simulink model "Battery_model"  (R2023b)
settings: Solver=FixedStepDiscrete  StartTime=0.0  StopTime=30000  RelTol=1e-3
values from neighbouring files (symbols this model uses):
  cf = 17e-6    (= 1.7e-05)    [Parameters.m]
  Kii_d = 100    [Parameters.m]
  Kii_dc = 0.003    [Parameters.m]
  Kii_q = 100    [Parameters.m]
  Kiv_dc = 10    [Parameters.m]
  Kpi_d = 1    [Parameters.m]
  Kpi_dc = 0.1    [Parameters.m]
  Kpi_q = 1    [Parameters.m]
  Kpv_dc = 30    [Parameters.m]
  lf = 1e-3    (= 0.001)    [Parameters.m]
  rf = 0    [Parameters.m]
  T_camp = 1    [Parameters.m]
  Ts_p = 80.0e-06    (= 8e-05)    [Parameters.m]
  Ts_Power = 80.0e-06    (= 8e-05)    [Parameters.m]
  V_ref_dc_link = 750    [Parameters.m]
undefined symbols (not defined in the file or in its folder): Ion, Lithium
libraries: spsRMSLib x9, spsThreePhaseVIMeasurementLib x5, slpidlib x4, spsabctodq0Lib x3, spsVoltageMeasurementLib x3, spsPower3phInstantaneousLib x3, spsPLLLib x3, spsTHDLib x3, simulink x2, spsCurrentMeasurementLib x2, spsThreePhaseSeriesRLCBranchLib x2, spsBatteryLib x1
settings Model: SimulationMode=accelerator  Creator=robby  LastModifiedBy=alessandroarmellin
settings SolverCC: AlgebraicLoopSolver=TrustRegion
settings DataIOCC: InitialState=out.xFinal  SaveFinalState=on  SaveOperatingPoint=on
settings ModelReferenceCC: EnableRefExpFcnMdlSchedulingChecks=on
settings RTWCC: DLArmComputeVersion=19.05

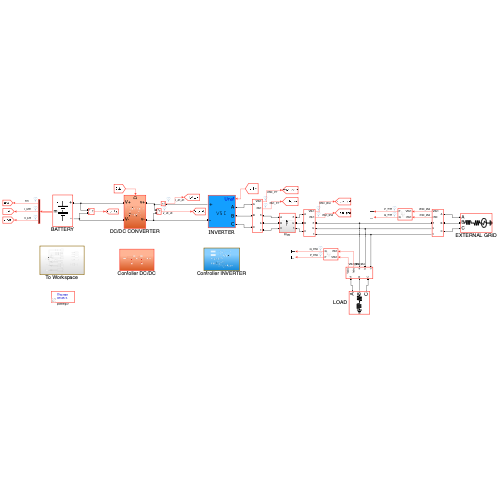
[thumbnail: Simulink's stored preview of the top-level diagram]
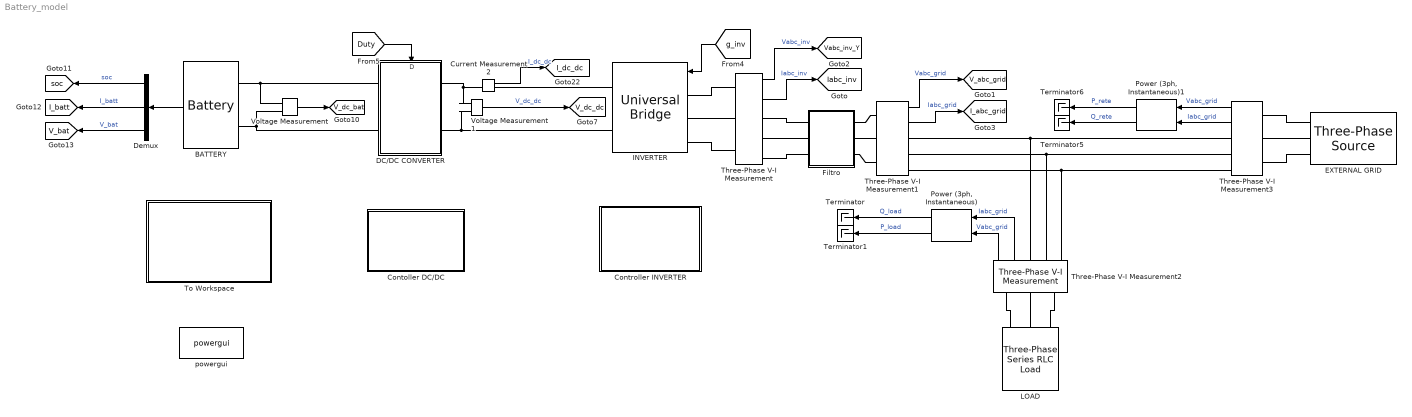
== system Battery_model ==
  BATTERY : spsBatteryLib/Battery  BatType=Lithium-Ion  ShowTempParam=off  ThermalPreset=no  ShowAgeParam=off  NomV=V_batt_nom  NomQ=Cap_bat_nom  SOC=soc_tot  Batt_Tr=1  PresetModel=on  MaxQ=200  MinV=465  FullV=721.672  Dis_rate=86.9565  R=0.031  Normal_OP=180.8696  expZone="[669.8392      9.826087]"  current=[6.5 13 32.5]  Units=Time  Tci=20  NomT=20  T2=-30  MaxQ2=4.8  FullV2=7.1  Normal_OP2=5.655  expZone2="[6.58           1]"  Rca=0.6  ti=2000  Dp=0  Neq0=0  Tsim=1e6  Ta1=25  Qeol=5.4*0.9  Reol=0.013333*1.2  Char_age=[2.3478, 3]  Dis_age=[2.3478, 10]  N1=1500  N2=10500  N3=1000  N4=1400  Ta2=45  N5=950
  Contoller DC/DC : Subsystem
  Controller INVERTER : Subsystem
  Current Measurement2 : spsCurrentMeasurementLib/Current Measurement  PhasorSimulation=off  OutputType=Complex  PSBequivalent=0
  DC/DC CONVERTER : Subsystem
      settings: PortSchema="{\"entries\":[{\"content\":{\"sides\":[{\"content\":{\"connectorIds\":[\"LConn1\",\"LConn2\"]},\"type\":\"ConnectorPlacement.EquallySpacedRectSide\",\"uuid\":\"1063a80c-0db9-4e6a-b0a1-ad7a8a9cb9ed\"},{\"content\":{\"connectorIds\":[\"RConn1\",\"RConn2\"],\"side\":\"RIGHT\"},\"type\":\"ConnectorPlacement.EquallySpacedRectSide\",\"uuid\":\"d09a7538-6c2e-450d-96ff-912ee6979d92\"},{\"content\":{\"connectorIds\":[\"In1\"],\"side\":\"TOP\"},\"type\":\"ConnectorPlacement.EquallySpacedRectSide\",\"uuid\":\"7f294bc1-8c9a-4b69-a306-35098527c416\"},{\"content\":{\"connectorIds\":[],\"side\":\"HIDDEN\"},\"type\":\"ConnectorPlacement.EquallySpacedRectSide\",\"uuid\":\"5677a460-882c-466a-84c4-3fc7d1866fb0\"}]},\"type\":\"ConnectorPlacement.EquallySpacedConnector\",\"uuid\":\"dc710a20-86db-486e-80ec-dfab0fa59d77\"}],\"packageUris\":[\"http://schema.mathworks.com/mf0/Connector/R2020b\"],\"version\":\"1.0\"}"
  Demux : Demux  Outputs=3
  EXTERNAL GRID : spsThreePhaseSourceLib/Three-Phase Source  InternalConnection=Yg  VoltagePhases=off  Voltage=400  PhaseAngle=0  Voltage_phases=[25e3 25e3 25e3]/sqrt(3)  PhaseAngles_phases=[0 -120 +120]  Frequency=50  NonIdealSource=on  SpecifyImpedance=off  Resistance=0.1  Inductance=1e-6  ShortCircuitLevel=1e6  BaseVoltage=400  XRratio=7  BusType=swing  Pref=10e3  Qref=0  Prefabc=[10e3, 10e3, 10e3]  Qrefabc=[0, 0, 0]  Qmin=-inf  Qmax=inf
  Filtro : Subsystem
  INVERTER : spsUniversalBridgeLib/Universal Bridge  Arms=3  SnubberResistance=1e5  SnubberCapacitance=inf  Device=Average-model based VSC  Ron=1e-3  Lon=0  ForwardVoltages="[  0  0  ]"  ForwardVoltage=0  GTOparameters=[ 10e-6 , 20e-6 ]  IGBTparameters=[ 1e-6 , 2e-6 ]  Measurements=None  Measurements_2=None  converterType=Rectifier
  LOAD : spsThreePhaseSeriesRLCLoadLib/Three-Phase Series RLC Load  LConnTagsString=A|B|C  Configuration=Y (grounded)  NominalVoltage=400  Vabc=[1e3 1e3 1e3]  Vabcp=[1e3 1e3 1e3]  NominalFrequency=50  UnbalancedPower=off  ActivePower=2000  InductivePower=150  CapacitivePower=0  Pabc=[10e3 9e3 11e3]  QLabc=[100 90 110]  QCabc=[100 90 110]  Pabcp=[10e3 9e3 11e3]  QLabcp=[100 90 110]  QCabcp=[100 90 110]  Measurements=None  LoadType=constant Z
  "Power (3ph, Instantaneous)" : spsPower3phInstantaneousLib/Power (3ph, Instantaneous)
  "Power (3ph, Instantaneous)1" : spsPower3phInstantaneousLib/Power (3ph, Instantaneous)
  Terminator{,1,5..6} (4 alike) : Terminator
  Three-Phase V-I Measurement{,1..3} (4 alike) : spsThreePhaseVIMeasurementLib/Three-Phase V-I Measurement  VoltageMeasurement=phase-to-ground  SetLabelV=off  LabelV=Vabc_cond  Vpu=off  VpuLL=off  CurrentMeasurement=yes  SetLabelI=off  LabelI=Iabc_cond  Ipu=off  Pbase=100e6  Vbase=500e3  OutputType=Complex  PhasorSimulation=off  PSBequivalent=0
  To Workspace : Subsystem
  Voltage Measurement : spsVoltageMeasurementLib/Voltage Measurement  PhasorSimulation=off  OutputType=Complex  PSBequivalent=0
  Voltage Measurement1 : spsVoltageMeasurementLib/Voltage Measurement  PhasorSimulation=off  OutputType=Complex  PSBequivalent=0
  powergui : spspowerguiLib/powergui  Priority=1  SimulationMode=Discrete  SampleTime=Ts_Power  frequency=60  Iterations=50  frequencyindice=50  Pbase=100e6  ErrMax=1e-4  UnitsV=kV  UnitsW=MW  buscounter=1  FunctionMessages=off  echomessages=off  EnableUseOfTLC=off  CurrentSourceSwitches=off  DisableSnubberDevices=off  DisableRonSwitches=off  DisableVfSwitches=off  DisplayEquations=off  AutomaticDiscreteSolvers=off  SolverType=Tustin/Backward Euler (TBE)  Interpol=off  ExternalGateDelay=off  methode=off  Ts=100  x0status=blocks  SPID=on  SwTol=0  HookPort=off  NonlinearTolerance=1e-4  nMaxIteration=100  ContinueOnMaxIteration=off  RestoreLinks=warning  ResistiveCurrentMeasurement=off  Frange=[0:2:500]  Ylog=off  Xlog=on  ShowGrid=off  save=off  variable=ZData  structure=0  ZoomFFT=off  StartTime=0.0  cycles=1  DisplayStyle=1  fundamental=60  FreqAxis=off  MaxFrequency=1000  frequencyindicesteady=1  RmsSteady=1  display=off
  tag scope: I_abc_grid=global, I_batt=global, I_dc_dc=global, Iabc_inv=global, V_abc_grid=global, V_bat=global, V_dc_bat=global, V_dc_dc=global, Vabc_inv_Y=global, soc=global
  wires:
  Three-Phase V-I Measurement/1 -> [Vabc_inv_Y]  "Vabc_inv"
  Three-Phase V-I Measurement/2 -> [Iabc_inv]  "Iabc_inv"
  Voltage Measurement1/1 -> [V_dc_dc]  "V_dc_dc"
  Current Measurement2/1 -> [I_dc_dc]  "I_dc_dc"
  [g_inv] -> INVERTER/1
  [Duty] -> DC/DC CONVERTER/1(D)
  BATTERY/1 -> Demux/1
  Demux/1 -> [soc]  "soc"
  Demux/2 -> [I_batt]  "I_batt"
  Demux/3 -> [V_bat]  "V_bat"
  Three-Phase V-I Measurement1/1 -> [V_abc_grid]  "Vabc_grid"
  Three-Phase V-I Measurement1/2 -> [I_abc_grid]  "Iabc_grid"
  Voltage Measurement/1 -> [V_dc_bat]
  Three-Phase V-I Measurement2/1 -> "Power (3ph, Instantaneous)"/1  "Vabc_grid"
  Three-Phase V-I Measurement2/2 -> "Power (3ph, Instantaneous)"/2  "Iabc_grid"
  "Power (3ph, Instantaneous)"/2 -> Terminator/1  "Q_load"
  "Power (3ph, Instantaneous)"/1 -> Terminator1/1  "P_load"
  "Power (3ph, Instantaneous)1"/1 -> Terminator6/1  "P_rete"
  "Power (3ph, Instantaneous)1"/2 -> Terminator5/1  "Q_rete"
  Three-Phase V-I Measurement3/2 -> "Power (3ph, Instantaneous)1"/2  "Iabc_grid"
  Three-Phase V-I Measurement3/1 -> "Power (3ph, Instantaneous)1"/1  "Vabc_grid"
  connections:
  Three-Phase V-I Measurement/LConn3 -- INVERTER/LConn3
  Three-Phase V-I Measurement/LConn2 -- INVERTER/LConn2
  Current Measurement2/RConn1 -- INVERTER/RConn1
  Current Measurement2/LConn1 -- Voltage Measurement1/LConn1 -- DC/DC CONVERTER/RConn1
  Voltage Measurement1/LConn2 -- INVERTER/RConn2 -- DC/DC CONVERTER/RConn2
  BATTERY/LConn1 -- Voltage Measurement/LConn1 -- DC/DC CONVERTER/LConn1
  Voltage Measurement/LConn2 -- BATTERY/LConn2 -- DC/DC CONVERTER/LConn2
  Filtro/LConn3 -- Three-Phase V-I Measurement/RConn3
  Filtro/LConn2 -- Three-Phase V-I Measurement/RConn2
  Filtro/LConn1 -- Three-Phase V-I Measurement/RConn1
  INVERTER/LConn1 -- Three-Phase V-I Measurement/LConn1
  Three-Phase V-I Measurement1/RConn2 -- Three-Phase V-I Measurement3/RConn2 -- Three-Phase V-I Measurement2/RConn2
  Three-Phase V-I Measurement2/RConn1 -- Three-Phase V-I Measurement1/RConn1 -- Three-Phase V-I Measurement3/RConn1
  Three-Phase V-I Measurement2/RConn3 -- Three-Phase V-I Measurement1/RConn3 -- Three-Phase V-I Measurement3/RConn3
  Three-Phase V-I Measurement1/LConn2 -- Filtro/RConn2
  Three-Phase V-I Measurement1/LConn3 -- Filtro/RConn3
  Filtro/RConn1 -- Three-Phase V-I Measurement1/LConn1
  Three-Phase V-I Measurement2/LConn2 -- LOAD/LConn2
  Three-Phase V-I Measurement2/LConn1 -- LOAD/LConn1
  Three-Phase V-I Measurement2/LConn3 -- LOAD/LConn3
  EXTERNAL GRID/RConn2 -- Three-Phase V-I Measurement3/LConn2
  Three-Phase V-I Measurement3/LConn1 -- EXTERNAL GRID/RConn1
  Three-Phase V-I Measurement3/LConn3 -- EXTERNAL GRID/RConn3

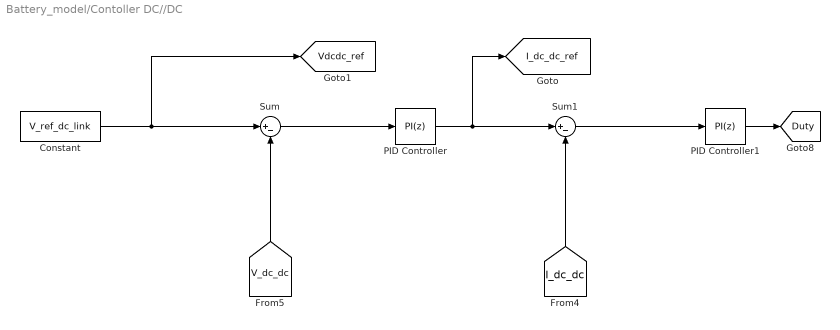
== system Battery_model/Contoller DC//DC ==
  Constant : Constant  Value=V_ref_dc_link
  PID Controller : slpidlib/PID Controller  Controller=PI  Form=Parallel  TimeDomain=Discrete-time  UseExternalTs=off  SampleTime=Ts_p  IntegratorMethod=Forward Euler  FilterMethod=Forward Euler  ControllerParametersSource=internal  P=Kiv_dc  I=Kpv_dc  UseKiTs=off  D=0  N=100  UseFilter=on  TunerSelectOption=Transfer Function Based (PID Tuner App)  InitialConditionSource=internal  InitialConditionForIntegrator=0  InitialConditionForFilter=0  DifferentiatorICPrevScaledInput=0  ExternalReset=none  TrackingMode=off  Kt=1  LimitOutput=off  SatLimitsSource=internal  UpperSaturationLimit=1  LowerSaturationLimit=-1  LinearizeAsGain=on  AntiWindupMode=none  Kb=1  LimitIntegrator=off  UpperIntegratorSaturationLimit=inf  LowerIntegratorSaturationLimit=-inf  POutMin=[]  POutMax=[]  IOutMin=[]  IOutMax=[]  DOutMin=[]  DOutMax=[]  NOutMin=[]  NOutMax=[]  SumOutMin=[]  SumOutMax=[]  SaturationOutMin=[]  SaturationOutMax=[]  PParamMin=[]  PParamMax=[]  IParamMin=[]  IParamMax=[]  DParamMin=[]  DParamMax=[]  NParamMin=[]  NParamMax=[]  KbParamMin=[]  KbParamMax=[]  KtParamMin=[]  KtParamMax=[]  KbOutMin=[]  KbOutMax=[]  KtOutMin=[]  KtOutMax=[]  IntegratorOutMin=[]  IntegratorOutMax=[]  FilterOutMin=[]  FilterOutMax=[]  SumI1OutMin=[]  SumI1OutMax=[]  SumI2OutMin=[]  SumI2OutMax=[]  SumI3OutMin=[]  SumI3OutMax=[]  SumI4OutMin=[]  SumI4OutMax=[]  SumDOutMin=[]  SumDOutMax=[]  DifferentiatorOutMin=[]  DifferentiatorOutMax=[]  FilterDiffOutCoefMin=[]  FilterDiffOutCoefMax=[]  ReciprocalOutMin=[]  ReciprocalOutMax=[]  SumDenOutMin=[]  SumDenOutMax=[]  SumNumOutMin=[]  SumNumOutMax=[]  DivideOutMin=[]  DivideOutMax=[]  UdiffTsProdOutMin=[]  UdiffTsProdOutMax=[]  NTsProdOutMin=[]  NTsProdOutMax=[]  UintegralTsProdOutMin=[]  UintegralTsProdOutMax=[]  UngainTsProdOutMin=[]  UngainTsProdOutMax=[]  ClampingZeroOutDataTypeStr=Inherit: Inherit via back propagation  ClampingZeroOutMin=[]  ClampingZeroOutMax=[]  FilterDenConstantOutDataTypeStr=Inherit: Inherit via back propagation  FilterDenConstantOutMin=[]  FilterDenConstantOutMax=[]  PCopyOutDataTypeStr=Inherit: Inherit via back propagation  PCopyOutMin=[]  PCopyOutMax=[]  NCopyOutDataTypeStr=Inherit: Inherit via back propagation  NCopyOutMin=[]  NCopyOutMax=[]  IntegratorContinuousStateAttributes=''  IntegratorStateMustResolveToSignalObject=off  IntegratorRTWStateStorageClass=Auto  FilterContinuousStateAttributes=''  FilterStateMustResolveToSignalObject=off  FilterRTWStateStorageClass=Auto  ParallelPVariant=InternalParameters  IdealPVariant=Disabled  IVariant=InternalParameters  DVariant=Disabled  IntegratorVariant=Discrete  SatVariant=Disabled  AWVariant=Passthrough  PCopyVariant=Disabled  TRVariant=Disabled  FdbkBlocksVariant=Forward  IdealPFdbkVariant=Disabled  SatFdbkVariant=Disabled  DerivativeFilterVariant=Disabled  NVariant=Disabled  NCopyVariant=Disabled_SignalSpec  FilterICVariant=Disabled  IntegratorICVariant=InternalICs  ExternalResetVariant=Disabled  TRSumVariant=Passthrough  SumFdbkVariant=Disabled  SumVariant=Sum_PI  TsampFilterVariant=InternalTs  TsampNgainVariant=Passthrough  TsampIntegralVariant=Disabled_SignalSpec  ExternalSaturationOutDataTypeStr=Inherit: Same as second input
  PID Controller1 : slpidlib/PID Controller  Controller=PI  Form=Parallel  TimeDomain=Discrete-time  UseExternalTs=off  SampleTime=Ts_p  IntegratorMethod=Forward Euler  FilterMethod=Forward Euler  ControllerParametersSource=internal  P=Kii_dc  I=Kpi_dc  UseKiTs=off  D=0  N=100  UseFilter=on  TunerSelectOption=Transfer Function Based (PID Tuner App)  InitialConditionSource=internal  InitialConditionForIntegrator=0  InitialConditionForFilter=0  DifferentiatorICPrevScaledInput=0  ExternalReset=none  TrackingMode=off  Kt=1  LimitOutput=off  SatLimitsSource=internal  UpperSaturationLimit=1  LowerSaturationLimit=-1  LinearizeAsGain=on  AntiWindupMode=none  Kb=1  LimitIntegrator=off  UpperIntegratorSaturationLimit=inf  LowerIntegratorSaturationLimit=-inf  POutMin=[]  POutMax=[]  IOutMin=[]  IOutMax=[]  DOutMin=[]  DOutMax=[]  NOutMin=[]  NOutMax=[]  SumOutMin=[]  SumOutMax=[]  SaturationOutMin=[]  SaturationOutMax=[]  PParamMin=[]  PParamMax=[]  IParamMin=[]  IParamMax=[]  DParamMin=[]  DParamMax=[]  NParamMin=[]  NParamMax=[]  KbParamMin=[]  KbParamMax=[]  KtParamMin=[]  KtParamMax=[]  KbOutMin=[]  KbOutMax=[]  KtOutMin=[]  KtOutMax=[]  IntegratorOutMin=[]  IntegratorOutMax=[]  FilterOutMin=[]  FilterOutMax=[]  SumI1OutMin=[]  SumI1OutMax=[]  SumI2OutMin=[]  SumI2OutMax=[]  SumI3OutMin=[]  SumI3OutMax=[]  SumI4OutMin=[]  SumI4OutMax=[]  SumDOutMin=[]  SumDOutMax=[]  DifferentiatorOutMin=[]  DifferentiatorOutMax=[]  FilterDiffOutCoefMin=[]  FilterDiffOutCoefMax=[]  ReciprocalOutMin=[]  ReciprocalOutMax=[]  SumDenOutMin=[]  SumDenOutMax=[]  SumNumOutMin=[]  SumNumOutMax=[]  DivideOutMin=[]  DivideOutMax=[]  UdiffTsProdOutMin=[]  UdiffTsProdOutMax=[]  NTsProdOutMin=[]  NTsProdOutMax=[]  UintegralTsProdOutMin=[]  UintegralTsProdOutMax=[]  UngainTsProdOutMin=[]  UngainTsProdOutMax=[]  ClampingZeroOutDataTypeStr=Inherit: Inherit via back propagation  ClampingZeroOutMin=[]  ClampingZeroOutMax=[]  FilterDenConstantOutDataTypeStr=Inherit: Inherit via back propagation  FilterDenConstantOutMin=[]  FilterDenConstantOutMax=[]  PCopyOutDataTypeStr=Inherit: Inherit via back propagation  PCopyOutMin=[]  PCopyOutMax=[]  NCopyOutDataTypeStr=Inherit: Inherit via back propagation  NCopyOutMin=[]  NCopyOutMax=[]  IntegratorContinuousStateAttributes=''  IntegratorStateMustResolveToSignalObject=off  IntegratorRTWStateStorageClass=Auto  FilterContinuousStateAttributes=''  FilterStateMustResolveToSignalObject=off  FilterRTWStateStorageClass=Auto  ParallelPVariant=InternalParameters  IdealPVariant=Disabled  IVariant=InternalParameters  DVariant=Disabled  IntegratorVariant=Discrete  SatVariant=Disabled  AWVariant=Passthrough  PCopyVariant=Disabled  TRVariant=Disabled  FdbkBlocksVariant=Forward  IdealPFdbkVariant=Disabled  SatFdbkVariant=Disabled  DerivativeFilterVariant=Disabled  NVariant=Disabled  NCopyVariant=Disabled_SignalSpec  FilterICVariant=Disabled  IntegratorICVariant=InternalICs  ExternalResetVariant=Disabled  TRSumVariant=Passthrough  SumFdbkVariant=Disabled  SumVariant=Sum_PI  TsampFilterVariant=InternalTs  TsampNgainVariant=Passthrough  TsampIntegralVariant=Disabled_SignalSpec  ExternalSaturationOutDataTypeStr=Inherit: Same as second input
  Sum : Sum  Inputs=|+-
  Sum1 : Sum  Inputs=|+-
  tag scope: Duty=global, I_dc_dc_ref=global, Vdcdc_ref=global
  wires:
  PID Controller1/1 -> [Duty]
  Sum/1 -> PID Controller/1
  Sum1/1 -> PID Controller1/1
  Constant/1 -> Sum/1, [Vdcdc_ref]
  PID Controller/1 -> Sum1/1, [I_dc_dc_ref]
  [V_dc_dc] -> Sum/2
  [I_dc_dc] -> Sum1/2

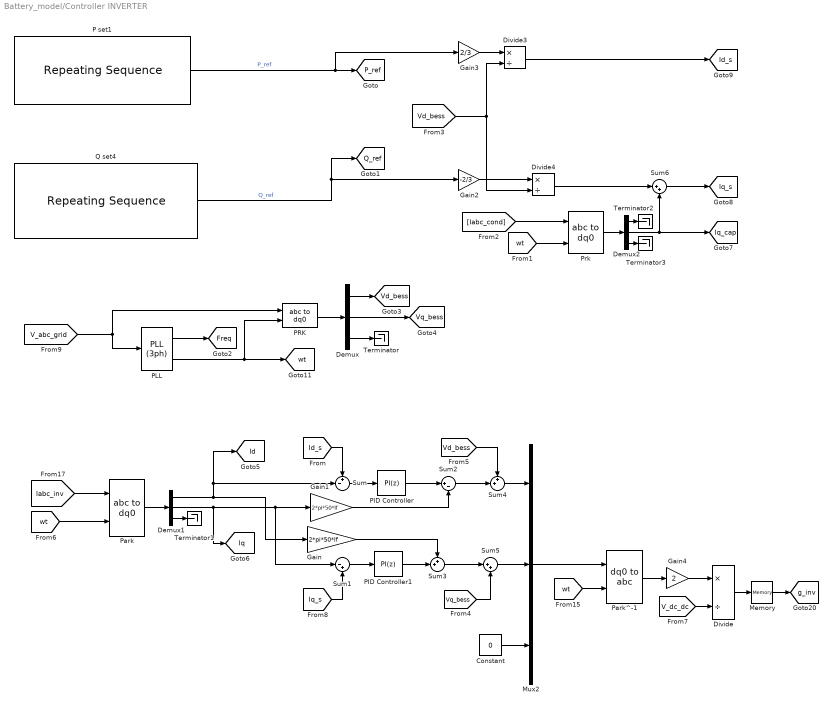
== system Battery_model/Controller INVERTER ==
  Constant : Constant  Value=0
  Demux : Demux  Outputs=3
  Demux1 : Demux  Outputs=3
  Demux2 : Demux  Outputs=3
  Divide : Product  Inputs=*/
  Divide3 : Product  Inputs=*/
  Divide4 : Product  Inputs=*/
  Gain : Gain  Gain=2*pi*50*lf
  Gain1 : Gain  Gain=2*pi*50*lf
  Gain2 : Gain  Gain=-2/3
  Gain3 : Gain  Gain=2/3
  Gain4 : Gain  Gain=2
  Memory : Memory  InitialCondition=0.1  InheritSampleTime=on
  Mux2 : Mux  Inputs=3
  P set1 : simulink/Sources/Repeating Sequence  rep_seq_t=[0 1 10 3610 3620 7220 7230 14430 14440 15040 15050 22250 22260 24060 24070 27670 27780 29480 29490 30000]  rep_seq_y=[0 0 40000 40000 20000 20000 10000 10000 0 0 -20000 -20000 -40000 -40000 -15000 -15000 -10000 -10000 0 0]
  PID Controller : slpidlib/PID Controller  Controller=PI  Form=Parallel  TimeDomain=Discrete-time  UseExternalTs=off  SampleTime=Ts_p  IntegratorMethod=Forward Euler  FilterMethod=Forward Euler  ControllerParametersSource=internal  P=Kpi_d  I=Kii_d  UseKiTs=off  D=0  N=100  UseFilter=on  TunerSelectOption=Transfer Function Based (PID Tuner App)  InitialConditionSource=internal  InitialConditionForIntegrator=0  InitialConditionForFilter=0  DifferentiatorICPrevScaledInput=0  ExternalReset=none  TrackingMode=off  Kt=1  LimitOutput=off  SatLimitsSource=internal  UpperSaturationLimit=inf  LowerSaturationLimit=-inf  LinearizeAsGain=on  AntiWindupMode=none  Kb=1  LimitIntegrator=off  UpperIntegratorSaturationLimit=inf  LowerIntegratorSaturationLimit=-inf  POutMin=[]  POutMax=[]  IOutMin=[]  IOutMax=[]  DOutMin=[]  DOutMax=[]  NOutMin=[]  NOutMax=[]  SumOutMin=[]  SumOutMax=[]  SaturationOutMin=[]  SaturationOutMax=[]  PParamMin=[]  PParamMax=[]  IParamMin=[]  IParamMax=[]  DParamMin=[]  DParamMax=[]  NParamMin=[]  NParamMax=[]  KbParamMin=[]  KbParamMax=[]  KtParamMin=[]  KtParamMax=[]  KbOutMin=[]  KbOutMax=[]  KtOutMin=[]  KtOutMax=[]  IntegratorOutMin=[]  IntegratorOutMax=[]  FilterOutMin=[]  FilterOutMax=[]  SumI1OutMin=[]  SumI1OutMax=[]  SumI2OutMin=[]  SumI2OutMax=[]  SumI3OutMin=[]  SumI3OutMax=[]  SumI4OutMin=[]  SumI4OutMax=[]  SumDOutMin=[]  SumDOutMax=[]  DifferentiatorOutMin=[]  DifferentiatorOutMax=[]  FilterDiffOutCoefMin=[]  FilterDiffOutCoefMax=[]  ReciprocalOutMin=[]  ReciprocalOutMax=[]  SumDenOutMin=[]  SumDenOutMax=[]  SumNumOutMin=[]  SumNumOutMax=[]  DivideOutMin=[]  DivideOutMax=[]  UdiffTsProdOutMin=[]  UdiffTsProdOutMax=[]  NTsProdOutMin=[]  NTsProdOutMax=[]  UintegralTsProdOutMin=[]  UintegralTsProdOutMax=[]  UngainTsProdOutMin=[]  UngainTsProdOutMax=[]  ClampingZeroOutDataTypeStr=Inherit: Inherit via back propagation  ClampingZeroOutMin=[]  ClampingZeroOutMax=[]  FilterDenConstantOutDataTypeStr=Inherit: Inherit via back propagation  FilterDenConstantOutMin=[]  FilterDenConstantOutMax=[]  PCopyOutDataTypeStr=Inherit: Inherit via back propagation  PCopyOutMin=[]  PCopyOutMax=[]  NCopyOutDataTypeStr=Inherit: Inherit via back propagation  NCopyOutMin=[]  NCopyOutMax=[]  IntegratorContinuousStateAttributes=''  IntegratorStateMustResolveToSignalObject=off  IntegratorRTWStateStorageClass=Auto  FilterContinuousStateAttributes=''  FilterStateMustResolveToSignalObject=off  FilterRTWStateStorageClass=Auto  ParallelPVariant=InternalParameters  IdealPVariant=Disabled  IVariant=InternalParameters  DVariant=Disabled  IntegratorVariant=Discrete  SatVariant=Disabled  AWVariant=Passthrough  PCopyVariant=Disabled  TRVariant=Disabled  FdbkBlocksVariant=Forward  IdealPFdbkVariant=Disabled  SatFdbkVariant=Disabled  DerivativeFilterVariant=Disabled  NVariant=Disabled  NCopyVariant=Disabled_SignalSpec  FilterICVariant=Disabled  IntegratorICVariant=InternalICs  ExternalResetVariant=Disabled  TRSumVariant=Passthrough  SumFdbkVariant=Disabled  SumVariant=Sum_PI  TsampFilterVariant=InternalTs  TsampNgainVariant=Passthrough  TsampIntegralVariant=Disabled_SignalSpec  ExternalSaturationOutDataTypeStr=Inherit: Same as second input
  PID Controller1 : slpidlib/PID Controller  Controller=PI  Form=Parallel  TimeDomain=Discrete-time  UseExternalTs=off  SampleTime=Ts_p  IntegratorMethod=Forward Euler  FilterMethod=Forward Euler  ControllerParametersSource=internal  P=Kpi_q  I=Kii_q  UseKiTs=off  D=0  N=100  UseFilter=on  TunerSelectOption=Transfer Function Based (PID Tuner App)  InitialConditionSource=internal  InitialConditionForIntegrator=0  InitialConditionForFilter=0  DifferentiatorICPrevScaledInput=0  ExternalReset=none  TrackingMode=off  Kt=1  LimitOutput=off  SatLimitsSource=internal  UpperSaturationLimit=inf  LowerSaturationLimit=-inf  LinearizeAsGain=on  AntiWindupMode=none  Kb=1  LimitIntegrator=off  UpperIntegratorSaturationLimit=inf  LowerIntegratorSaturationLimit=-inf  POutMin=[]  POutMax=[]  IOutMin=[]  IOutMax=[]  DOutMin=[]  DOutMax=[]  NOutMin=[]  NOutMax=[]  SumOutMin=[]  SumOutMax=[]  SaturationOutMin=[]  SaturationOutMax=[]  PParamMin=[]  PParamMax=[]  IParamMin=[]  IParamMax=[]  DParamMin=[]  DParamMax=[]  NParamMin=[]  NParamMax=[]  KbParamMin=[]  KbParamMax=[]  KtParamMin=[]  KtParamMax=[]  KbOutMin=[]  KbOutMax=[]  KtOutMin=[]  KtOutMax=[]  IntegratorOutMin=[]  IntegratorOutMax=[]  FilterOutMin=[]  FilterOutMax=[]  SumI1OutMin=[]  SumI1OutMax=[]  SumI2OutMin=[]  SumI2OutMax=[]  SumI3OutMin=[]  SumI3OutMax=[]  SumI4OutMin=[]  SumI4OutMax=[]  SumDOutMin=[]  SumDOutMax=[]  DifferentiatorOutMin=[]  DifferentiatorOutMax=[]  FilterDiffOutCoefMin=[]  FilterDiffOutCoefMax=[]  ReciprocalOutMin=[]  ReciprocalOutMax=[]  SumDenOutMin=[]  SumDenOutMax=[]  SumNumOutMin=[]  SumNumOutMax=[]  DivideOutMin=[]  DivideOutMax=[]  UdiffTsProdOutMin=[]  UdiffTsProdOutMax=[]  NTsProdOutMin=[]  NTsProdOutMax=[]  UintegralTsProdOutMin=[]  UintegralTsProdOutMax=[]  UngainTsProdOutMin=[]  UngainTsProdOutMax=[]  ClampingZeroOutDataTypeStr=Inherit: Inherit via back propagation  ClampingZeroOutMin=[]  ClampingZeroOutMax=[]  FilterDenConstantOutDataTypeStr=Inherit: Inherit via back propagation  FilterDenConstantOutMin=[]  FilterDenConstantOutMax=[]  PCopyOutDataTypeStr=Inherit: Inherit via back propagation  PCopyOutMin=[]  PCopyOutMax=[]  NCopyOutDataTypeStr=Inherit: Inherit via back propagation  NCopyOutMin=[]  NCopyOutMax=[]  IntegratorContinuousStateAttributes=''  IntegratorStateMustResolveToSignalObject=off  IntegratorRTWStateStorageClass=Auto  FilterContinuousStateAttributes=''  FilterStateMustResolveToSignalObject=off  FilterRTWStateStorageClass=Auto  ParallelPVariant=InternalParameters  IdealPVariant=Disabled  IVariant=InternalParameters  DVariant=Disabled  IntegratorVariant=Discrete  SatVariant=Disabled  AWVariant=Passthrough  PCopyVariant=Disabled  TRVariant=Disabled  FdbkBlocksVariant=Forward  IdealPFdbkVariant=Disabled  SatFdbkVariant=Disabled  DerivativeFilterVariant=Disabled  NVariant=Disabled  NCopyVariant=Disabled_SignalSpec  FilterICVariant=Disabled  IntegratorICVariant=InternalICs  ExternalResetVariant=Disabled  TRSumVariant=Passthrough  SumFdbkVariant=Disabled  SumVariant=Sum_PI  TsampFilterVariant=InternalTs  TsampNgainVariant=Passthrough  TsampIntegralVariant=Disabled_SignalSpec  ExternalSaturationOutDataTypeStr=Inherit: Same as second input
  PLL : spsPLL3phLib/PLL (3ph)  Fmin=45  Par_Init=[0, 50]  ParK=[180, 3200, 1]  TcD=1e-4  MaxRateChangeFreq=12  FilterCutOffFreq=25  Ts=Ts_p  AGC=on
  PRK : spsabctodq0Lib/abc to dq0  Alignment=90 degrees behind phase A axis
  Park : spsabctodq0Lib/abc to dq0  Alignment=90 degrees behind phase A axis
  Park^-1 : spsdq0toabcLib/dq0 to abc  Alignment=90 degrees behind phase A axis
  Prk : spsabctodq0Lib/abc to dq0  Alignment=90 degrees behind phase A axis
  Q set4 : simulink/Sources/Repeating Sequence  rep_seq_t=[0 1 10 3610 3620 7220 7230 14430 14440 15040 15050 22250 22260 24060 24070 27670 27780 29480 29490 30000]  rep_seq_y=[0 0 10000 10000 5000 5000 5000 5000 0 0 0 0 0 0 0 0 0 0 0 0]
  Sum : Sum  Inputs=+-|
  Sum1 : Sum  Inputs=|-+
  Sum2 : Sum  Inputs=|+-
  Sum3 : Sum  Inputs=++|
  Sum4 : Sum  Inputs=++|
  Sum5 : Sum  Inputs=|++
  Sum6 : Sum  Inputs=|++
  Terminator{,1..3} (4 alike) : Terminator
  tag scope: Freq=global, Id=global, Id_s=global, Iq=global, Iq_cap=global, Iq_s=global, P_ref=global, Q_ref=global, Vd_bess=global, Vq_bess=global, g_inv=global, wt=global
  wires:
  [Vq_bess] -> Sum5/2
  [Vd_bess] -> Sum4/1
  [Iq_s] -> Sum1/2
  [Id_s] -> Sum/1
  Gain1/1 -> Sum2/2
  PID Controller/1 -> Sum2/1
  PLL/1 -> [Freq]
  Demux/3 -> Terminator/1
  Sum3/1 -> Sum5/1
  PID Controller1/1 -> Sum3/2
  Demux/2 -> [Vq_bess]
  Gain/1 -> Sum3/1
  Demux/1 -> [Vd_bess]
  Constant/1 -> Mux2/3
  [wt] -> Park^-1/2
  Sum/1 -> PID Controller/1
  Sum4/1 -> Mux2/1
  Demux1/2 -> Sum1/1, Gain1/1, [Iq]
  Sum2/1 -> Sum4/2
  Demux1/1 -> [Id], Sum/2, Gain/1
  Demux1/3 -> Terminator1/1
  Sum1/1 -> PID Controller1/1
  Sum5/1 -> Mux2/2
  Park/1 -> Demux1/1
  PRK/1 -> Demux/1
  PLL/2 -> PRK/2, [wt]
  Divide4/1 -> Sum6/1
  [Vd_bess] -> Divide3/2, Divide4/2
  Gain2/1 -> Divide4/1
  Gain3/1 -> Divide3/1
  [wt] -> Prk/2
  Prk/1 -> Demux2/1
  Demux2/2 -> Sum6/2, [Iq_cap]
  Mux2/1 -> Park^-1/1
  Divide3/1 -> [Id_s]
  Sum6/1 -> [Iq_s]
  [Iabc_inv] -> Park/1
  [wt] -> Park/2
  [V_abc_grid] -> PLL/1, PRK/1
  [Iabc_cond] -> Prk/1
  Park^-1/1 -> Gain4/1
  Divide/1 -> Memory/1
  Gain4/1 -> Divide/1
  [V_dc_dc] -> Divide/2
  Memory/1 -> [g_inv]
  Demux2/3 -> Terminator3/1
  Demux2/1 -> Terminator2/1
  P set1/1 -> Gain3/1, [P_ref]  "P_ref"
  Q set4/1 -> Gain2/1, [Q_ref]  "Q_ref"

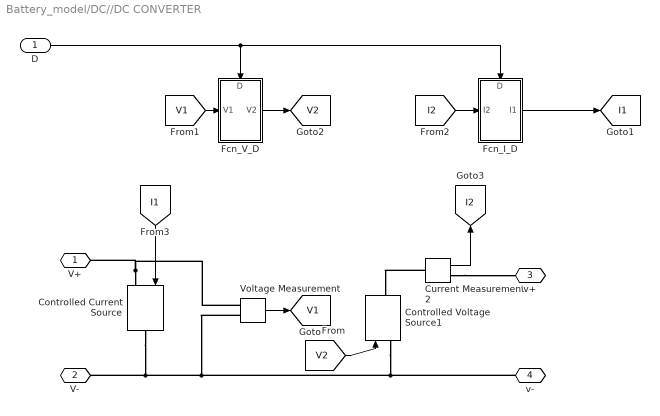
== system Battery_model/DC//DC CONVERTER ==
  D : Inport
  Controlled Current Source : spsControlledCurrentSourceLib/Controlled Current Source  Initialize=off  Source_Type=DC  Amplitude=0  Phase=0  Frequency=0  Measurements=None
  Controlled Voltage Source1 : spsControlledVoltageSourceLib/Controlled Voltage Source  Initialize=on  Source_Type=DC  Amplitude=0  Phase=0  Frequency=0  Measurements=None
  Current Measurement2 : spsCurrentMeasurementLib/Current Measurement  PhasorSimulation=off  OutputType=Complex  PSBequivalent=0
  Fcn_I_D : Subsystem
      settings: PortSchema="{\"entries\":[{\"content\":{\"sides\":[{\"content\":{\"connectorIds\":[\"In1\"]},\"type\":\"ConnectorPlacement.EquallySpacedRectSide\",\"uuid\":\"c3b5bf8f-c0a6-4eff-a00e-7fb1c6213418\"},{\"content\":{\"connectorIds\":[\"Out1\"],\"side\":\"RIGHT\"},\"type\":\"ConnectorPlacement.EquallySpacedRectSide\",\"uuid\":\"03805e13-a53e-47ff-ab0e-f9f14d4ce48a\"},{\"content\":{\"connectorIds\":[\"In2\"],\"side\":\"TOP\"},\"type\":\"ConnectorPlacement.EquallySpacedRectSide\",\"uuid\":\"bc21352b-7376-4339-9823-31e6d52a6fd4\"},{\"content\":{\"connectorIds\":[],\"side\":\"HIDDEN\"},\"type\":\"ConnectorPlacement.EquallySpacedRectSide\",\"uuid\":\"bc103710-efdf-4c70-addb-3237ca6c7db4\"}]},\"type\":\"ConnectorPlacement.EquallySpacedConnector\",\"uuid\":\"a5a32d25-b893-4253-b055-036b21e447f7\"}],\"packageUris\":[\"http://schema.mathworks.com/mf0/Connector/R2020b\"],\"version\":\"1.0\"}"
  Fcn_V_D : Subsystem
      settings: PortSchema="{\"entries\":[{\"content\":{\"sides\":[{\"content\":{\"connectorIds\":[\"In1\"]},\"type\":\"ConnectorPlacement.EquallySpacedRectSide\",\"uuid\":\"c3b5bf8f-c0a6-4eff-a00e-7fb1c6213418\"},{\"content\":{\"connectorIds\":[\"Out1\"],\"side\":\"RIGHT\"},\"type\":\"ConnectorPlacement.EquallySpacedRectSide\",\"uuid\":\"03805e13-a53e-47ff-ab0e-f9f14d4ce48a\"},{\"content\":{\"connectorIds\":[\"In2\"],\"side\":\"TOP\"},\"type\":\"ConnectorPlacement.EquallySpacedRectSide\",\"uuid\":\"bc21352b-7376-4339-9823-31e6d52a6fd4\"},{\"content\":{\"connectorIds\":[],\"side\":\"HIDDEN\"},\"type\":\"ConnectorPlacement.EquallySpacedRectSide\",\"uuid\":\"bc103710-efdf-4c70-addb-3237ca6c7db4\"}]},\"type\":\"ConnectorPlacement.EquallySpacedConnector\",\"uuid\":\"a5a32d25-b893-4253-b055-036b21e447f7\"}],\"packageUris\":[\"http://schema.mathworks.com/mf0/Connector/R2020b\"],\"version\":\"1.0\"}"
  Voltage Measurement : spsVoltageMeasurementLib/Voltage Measurement  PhasorSimulation=off  OutputType=Complex  PSBequivalent=0
  V+ : PMIOPort  Side=Left
  V- : PMIOPort  Port=2  Side=Left
  v+ : PMIOPort  Port=3  Side=Right
  v- : PMIOPort  Port=4  Side=Right
  tag scope: I1=global, I2=global, V1=global, V2=global
  wires:
  [V1] -> Fcn_V_D/1(V1)
  [V2] -> Controlled Voltage Source1/1
  [I1] -> Controlled Current Source/1
  [I2] -> Fcn_I_D/1(I2)
  Current Measurement2/1 -> [I2]
  Voltage Measurement/1 -> [V1]
  Fcn_V_D/1(V2) -> [V2]
  Fcn_I_D/1(I1) -> [I1]
  D/1 -> Fcn_V_D/2(D), Fcn_I_D/2(D)
  connections:
  v-/RConn1 -- Controlled Voltage Source1/LConn1 -- V-/RConn1 -- Controlled Current Source/RConn1 -- Voltage Measurement/LConn2
  Current Measurement2/RConn1 -- v+/RConn1
  Current Measurement2/LConn1 -- Controlled Voltage Source1/RConn1
  Controlled Current Source/LConn1 -- V+/RConn1 -- Voltage Measurement/LConn1

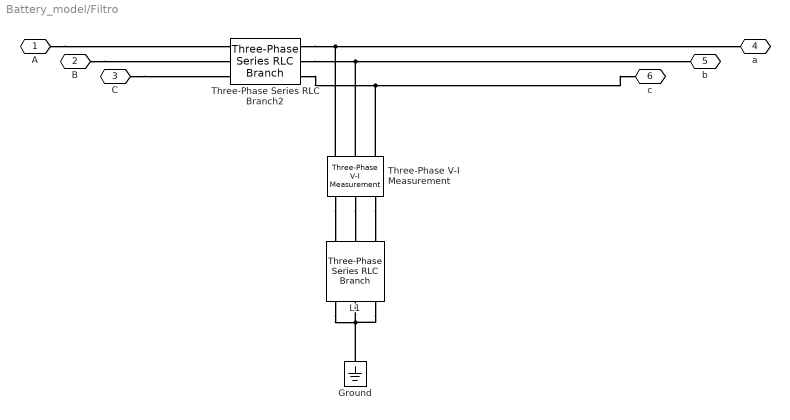
== system Battery_model/Filtro ==
  Ground : spsGroundLib/Ground  LConnTagsString=a
  L1 : spsThreePhaseSeriesRLCBranchLib/Three-Phase Series RLC Branch  LConnTagsString=A|B|C  RConnTagsString=A|B|C  BranchType=C  Resistance=0.02e-3  Inductance=0.08e-3  Capacitance=cf  Measurements=None
  Three-Phase Series RLC Branch2 : spsThreePhaseSeriesRLCBranchLib/Three-Phase Series RLC Branch  LConnTagsString=A|B|C  RConnTagsString=A|B|C  BranchType=L  Resistance=rf  Inductance=lf  Capacitance=1e-6  Measurements=None
  Three-Phase V-I Measurement : spsThreePhaseVIMeasurementLib/Three-Phase V-I Measurement  VoltageMeasurement=phase-to-ground  SetLabelV=on  LabelV=Vabc_cond  Vpu=off  VpuLL=off  CurrentMeasurement=yes  SetLabelI=on  LabelI=Iabc_cond  Ipu=off  Pbase=100e6  Vbase=500e3  OutputType=Complex  PhasorSimulation=off  PSBequivalent=0
  A : PMIOPort  Side=Left
  B : PMIOPort  Port=2  Side=Left
  C : PMIOPort  Port=3  Side=Left
  a : PMIOPort  Port=4  Side=Right
  b : PMIOPort  Port=5  Side=Right
  c : PMIOPort  Port=6  Side=Right
  connections:
  C/RConn1 -- Three-Phase Series RLC Branch2/LConn3
  B/RConn1 -- Three-Phase Series RLC Branch2/LConn2
  A/RConn1 -- Three-Phase Series RLC Branch2/LConn1
  L1/RConn1 -- L1/RConn3 -- Ground/LConn1 -- L1/RConn2
  Three-Phase Series RLC Branch2/RConn1 -- a/RConn1 -- Three-Phase V-I Measurement/LConn1
  Three-Phase Series RLC Branch2/RConn2 -- b/RConn1 -- Three-Phase V-I Measurement/LConn2
  Three-Phase Series RLC Branch2/RConn3 -- c/RConn1 -- Three-Phase V-I Measurement/LConn3
  Three-Phase V-I Measurement/RConn1 -- L1/LConn1
  Three-Phase V-I Measurement/RConn2 -- L1/LConn2
  Three-Phase V-I Measurement/RConn3 -- L1/LConn3

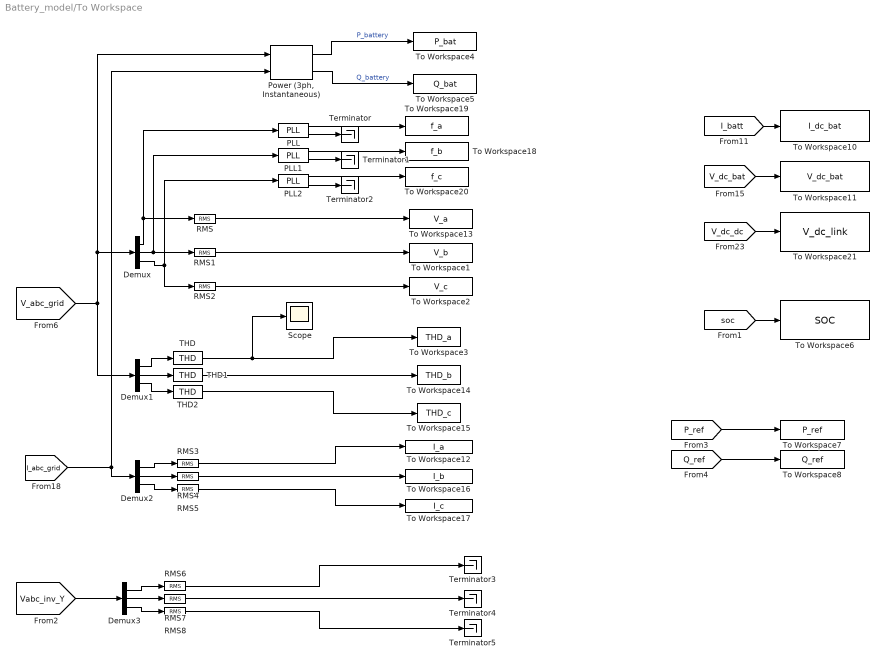
== system Battery_model/To Workspace ==
  Demux{,1..3} (4 alike) : Demux  Outputs=3
  PLL : spsPLLLib/PLL  Fmin=45  Par_Init=[0, 50]  ParK=[180, 3200, 1]  TcD=1e-4  MaxRateChangeFreq=12  FilterCutOffFreq=25  Ts=Ts_Power  AGC=on
  PLL1 : spsPLLLib/PLL  Fmin=45  Par_Init=[0, 50]  ParK=[180, 3200, 1]  TcD=1e-4  MaxRateChangeFreq=12  FilterCutOffFreq=25  Ts=Ts_Power  AGC=on
  PLL2 : spsPLLLib/PLL  Fmin=45  Par_Init=[0, 50]  ParK=[180, 3200, 1]  TcD=1e-4  MaxRateChangeFreq=12  FilterCutOffFreq=25  Ts=Ts_Power  AGC=on
  "Power (3ph, Instantaneous)" : spsPower3phInstantaneousLib/Power (3ph, Instantaneous)
  RMS{,1..8} (9 alike) : spsRMSLib/RMS  TrueRMS=on  Freq=50  RMSInit=400  Ts=Ts_Power
  Scope : Scope
  THD : spsTHDLib/THD  Freq=50  Ts=Ts_p
  THD1 : spsTHDLib/THD  Freq=50  Ts=Ts_p
  THD2 : spsTHDLib/THD  Freq=50  Ts=Ts_p
  Terminator{,1..5} (6 alike) : Terminator
  To Workspace1 : ToWorkspace  VariableName=V_b  SampleTime=T_camp
  To Workspace10 : ToWorkspace  VariableName=I_dc_bat  SampleTime=T_camp
  To Workspace11 : ToWorkspace  VariableName=V_dc_bat  SampleTime=T_camp
  To Workspace12 : ToWorkspace  VariableName=I_a  SampleTime=T_camp
  To Workspace13 : ToWorkspace  VariableName=V_a  SampleTime=T_camp
  To Workspace14 : ToWorkspace  VariableName=THD_b  SampleTime=T_camp
  To Workspace15 : ToWorkspace  VariableName=THD_c  SampleTime=T_camp
  To Workspace16 : ToWorkspace  VariableName=I_b  SampleTime=T_camp
  To Workspace17 : ToWorkspace  VariableName=I_c  SampleTime=T_camp
  To Workspace18 : ToWorkspace  VariableName=f_b  SampleTime=T_camp
  To Workspace19 : ToWorkspace  VariableName=f_a  SampleTime=T_camp
  To Workspace2 : ToWorkspace  VariableName=V_c  SampleTime=T_camp
  To Workspace20 : ToWorkspace  VariableName=f_c  SampleTime=T_camp
  To Workspace21 : ToWorkspace  VariableName=V_dc_link  SampleTime=T_camp
  To Workspace3 : ToWorkspace  VariableName=THD_a  SampleTime=T_camp
  To Workspace4 : ToWorkspace  VariableName=P_bat  SampleTime=T_camp
  To Workspace5 : ToWorkspace  VariableName=Q_bat  SampleTime=T_camp
  To Workspace6 : ToWorkspace  VariableName=SOC  SampleTime=T_camp
  To Workspace7 : ToWorkspace  VariableName=P_ref  SampleTime=T_camp
  To Workspace8 : ToWorkspace  VariableName=Q_ref  SampleTime=T_camp
  wires:
  [V_abc_grid] -> Demux/1, "Power (3ph, Instantaneous)"/1, Demux1/1
  [I_batt] -> To Workspace10/1
  [V_dc_bat] -> To Workspace11/1
  THD/1 -> Scope/1, To Workspace3/1
  Demux/2 -> RMS1/1, PLL1/1
  Demux/1 -> PLL/1, RMS/1
  Demux/3 -> PLL2/1, RMS2/1
  RMS/1 -> To Workspace13/1
  RMS1/1 -> To Workspace1/1
  RMS2/1 -> To Workspace2/1
  Demux1/1 -> THD/1
  Demux1/2 -> THD1/1
  Demux1/3 -> THD2/1
  THD1/1 -> To Workspace14/1
  THD2/1 -> To Workspace15/1
  Demux2/3 -> RMS5/1
  Demux2/1 -> RMS3/1
  Demux2/2 -> RMS4/1
  [I_abc_grid] -> "Power (3ph, Instantaneous)"/2, Demux2/1
  RMS3/1 -> To Workspace12/1
  RMS4/1 -> To Workspace16/1
  RMS5/1 -> To Workspace17/1
  PLL/2 -> Terminator/1
  PLL1/2 -> Terminator1/1
  PLL2/2 -> Terminator2/1
  PLL2/1 -> To Workspace20/1
  PLL1/1 -> To Workspace18/1
  PLL/1 -> To Workspace19/1
  [V_dc_dc] -> To Workspace21/1
  "Power (3ph, Instantaneous)"/1 -> To Workspace4/1  "P_battery"
  "Power (3ph, Instantaneous)"/2 -> To Workspace5/1  "Q_battery"
  [soc] -> To Workspace6/1
  [Vabc_inv_Y] -> Demux3/1
  Demux3/3 -> RMS8/1
  Demux3/2 -> RMS7/1
  Demux3/1 -> RMS6/1
  RMS7/1 -> Terminator4/1
  RMS6/1 -> Terminator3/1
  RMS8/1 -> Terminator5/1
  [Q_ref] -> To Workspace8/1
  [P_ref] -> To Workspace7/1

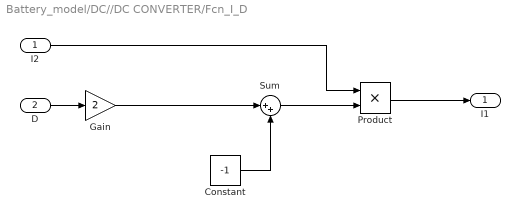
== system Battery_model/DC//DC CONVERTER/Fcn_I_D ==
  I2 : Inport
  D : Inport  Port=2
  Constant : Constant  Value=-1
  Gain : Gain  Gain=2
  Product : Product
  Sum : Sum  Inputs=|++
  I1 : Outport
  wires:
  Constant/1 -> Sum/2
  Sum/1 -> Product/2
  D/1 -> Gain/1
  Product/1 -> I1/1
  I2/1 -> Product/1
  Gain/1 -> Sum/1

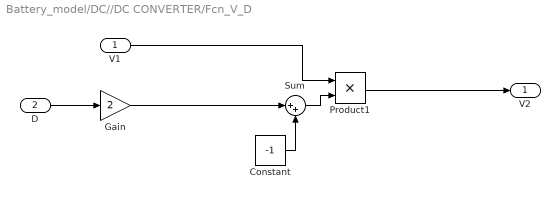
== system Battery_model/DC//DC CONVERTER/Fcn_V_D ==
  V1 : Inport
  D : Inport  Port=2
  Constant : Constant  Value=-1
  Gain : Gain  Gain=2
  Product1 : Product
  Sum : Sum  Inputs=|++
  V2 : Outport
  wires:
  Sum/1 -> Product1/2
  D/1 -> Gain/1
  Constant/1 -> Sum/2
  Product1/1 -> V2/1
  Gain/1 -> Sum/1
  V1/1 -> Product1/1
